simulink model "Brake_Signal_Model"  (R2024a)
settings: Solver=VariableStepAuto  StartTime=0.0  StopTime=inf  RelTol=1e-3
settings Model: Creator=ec97883  LastModifiedBy=ec97883

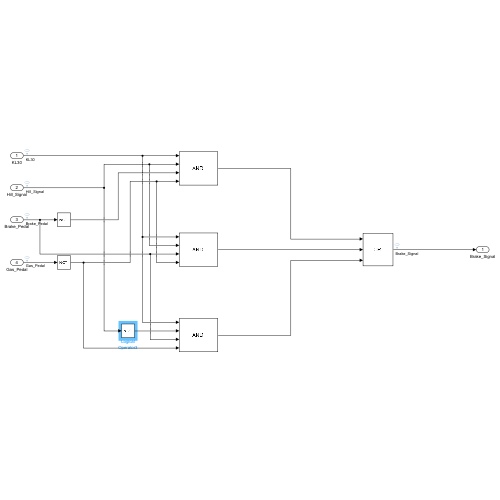
[thumbnail: Simulink's stored preview of the top-level diagram]
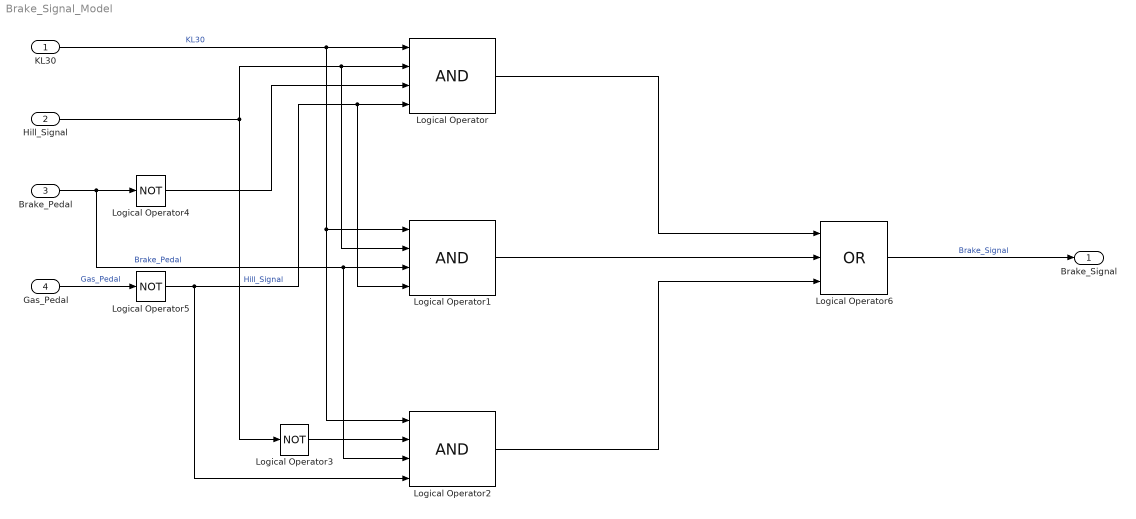
== system Brake_Signal_Model ==
  KL30 : Inport  OutDataTypeStr=boolean  PortDimensions=1
  Hill_Signal : Inport  Port=2  OutDataTypeStr=boolean  PortDimensions=1
  Brake_Pedal : Inport  Port=3  OutDataTypeStr=boolean  PortDimensions=1
  Gas_Pedal : Inport  Port=4  OutDataTypeStr=boolean  PortDimensions=1
  Logical Operator : Logic  Inputs=4  AllPortsSameDT=off  OutDataTypeStr=boolean
  Logical Operator1 : Logic  Inputs=4  AllPortsSameDT=off  OutDataTypeStr=boolean
  Logical Operator2 : Logic  Inputs=4  AllPortsSameDT=off  OutDataTypeStr=boolean
  Logical Operator3 : Logic  Operator=NOT  AllPortsSameDT=off  OutDataTypeStr=boolean
  Logical Operator4 : Logic  Operator=NOT  AllPortsSameDT=off  OutDataTypeStr=boolean
  Logical Operator5 : Logic  Operator=NOT  AllPortsSameDT=off  OutDataTypeStr=boolean
  Logical Operator6 : Logic  Operator=OR  Inputs=3  AllPortsSameDT=off  OutDataTypeStr=boolean
  Brake_Signal : Outport  OutDataTypeStr=boolean  PortDimensions=1
  wires:
  KL30/1 -> Logical Operator2/1, Logical Operator1/1, Logical Operator/1  "KL30"
  Hill_Signal/1 -> Logical Operator3/1, Logical Operator1/2, Logical Operator/2  "Hill_Signal"
  Brake_Pedal/1 -> Logical Operator2/3, Logical Operator1/3, Logical Operator4/1  "Brake_Pedal"
  Logical Operator4/1 -> Logical Operator/3
  Gas_Pedal/1 -> Logical Operator5/1  "Gas_Pedal"
  Logical Operator5/1 -> Logical Operator2/4, Logical Operator1/4, Logical Operator/4
  Logical Operator1/1 -> Logical Operator6/2
  Logical Operator/1 -> Logical Operator6/1
  Logical Operator2/1 -> Logical Operator6/3
  Logical Operator6/1 -> Brake_Signal/1  "Brake_Signal"
  Logical Operator3/1 -> Logical Operator2/2
